simulink model "FourTanks_PID"  (R2023b)
settings: Solver=ode4  StartTime=0.0  StopTime=1600  FixedStep=1/100  MinStep=0.01  RelTol=1e-3  EnableMultiTasking=on
InitFcn:
  | init_fourtanks
model workspace (MAT data in the model file):
  PID_params = [98.4128186329 97.7718380758 37.9597023931 70.0809402327 32.7398112273 96.4014930201]
values from neighbouring files (symbols this model uses):
  A1 = 28    [init_fourtanks.m]
  A2 = 32    [init_fourtanks.m]
  A3 = 28    [init_fourtanks.m]
  A4 = 32    [init_fourtanks.m]
  g = 981    [init_fourtanks.m]
  gamma1 = 0.7    [init_fourtanks.m]
  gamma2 = 0.7    [init_fourtanks.m]
  gamma3 = 1.0    (= 1)    [init_fourtanks.m]
  gamma4 = 1.0    (= 1)    [init_fourtanks.m]
  gammaA = 0.6    [init_fourtanks.m]
  gammaB = 0.6    [init_fourtanks.m]
  k1 = .071    (= 0.071)    [init_fourtanks.m]
  k2 = .057    (= 0.057)    [init_fourtanks.m]
  k3 = .071    (= 0.071)    [init_fourtanks.m]
  k4 = .057    (= 0.057)    [init_fourtanks.m]
  kA = 3.33    [init_fourtanks.m]
  kB = 3.35    [init_fourtanks.m]
undefined symbols (not defined in the file or in its folder): h, sigbuilder_block, u0
libraries: slpidlib x2
settings Model: Creator=Windows  LastModifiedBy=HP
settings SolverCC: AlgebraicLoopSolver=TrustRegion
settings OptimizationCC: DefaultParameterBehavior=Inlined  BufferReuse=off
settings DebuggingCC: UnconnectedInputMsg=warning  UnconnectedOutputMsg=warning  UnconnectedLineMsg=warning  InitInArrayFormatMsg=none  ArithmeticOperatorsInVariantConditions=warning
settings ModelReferenceCC: EnableRefExpFcnMdlSchedulingChecks=on
settings SFSimCC: CustomCodeUndefinedFunction=UseInterfaceOnly
settings RTWCC: DLArmComputeVersion=19.05

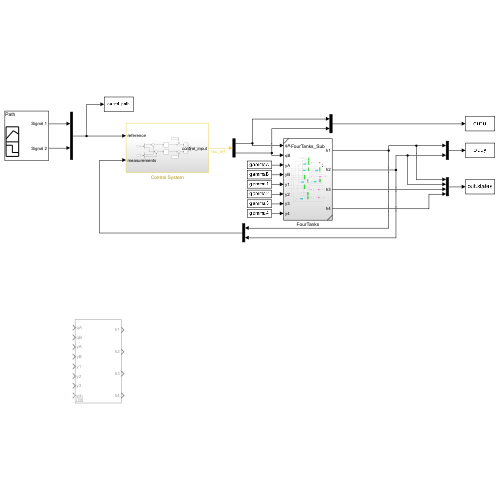
[thumbnail: Simulink's stored preview of the top-level diagram]
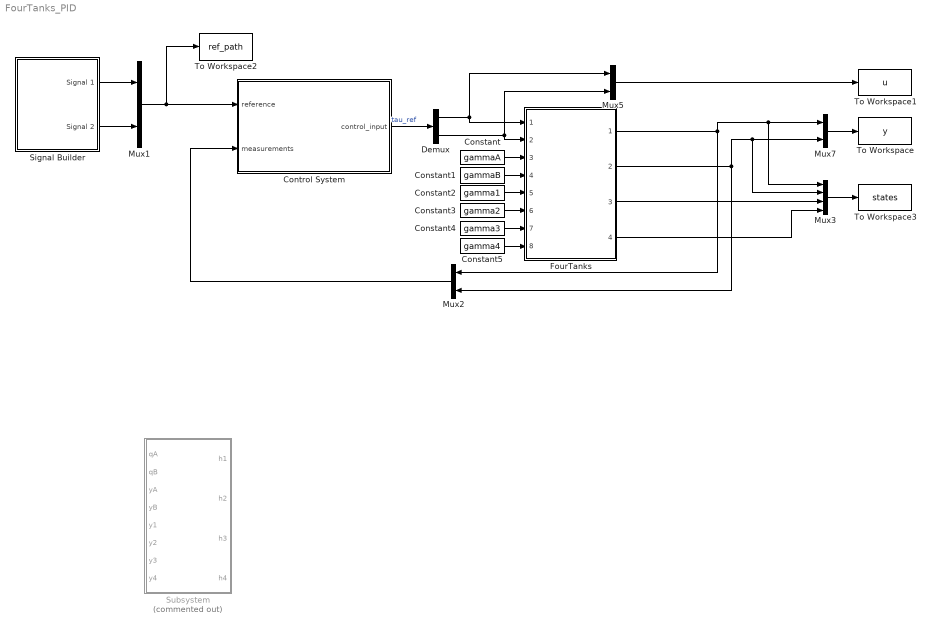
== system FourTanks_PID ==
  Constant : Constant  Value=gammaA
  Constant1 : Constant  Value=gammaB
  Constant2 : Constant  Value=gamma1
  Constant3 : Constant  Value=gamma2
  Constant4 : Constant  Value=gamma3
  Constant5 : Constant  Value=gamma4
  Control System : Subsystem
  Demux : Demux  Outputs=2
  FourTanks : Subsystem  ReferencedSubsystem=FourTanks_Sub
  Mux{1..2,5,7} (4 alike) : Mux  Inputs=2
  Mux3 : Mux
  Signal Builder : Subsystem  Tag=STV Subsys  LoadFcn=sigbuilder_block('load');  StartFcn=sigbuilder_block('start');  StopFcn=sigbuilder_block('stop');  ClipboardFcn=sigbuilder_block('clipboard');  mask(Sigbuilder block){tuvar=[0:10]}
      mask help: Simulink:masks:SigbuilderBlock_MD
      mask init:
      | if ~strcmp(get_param(bdroot(gcbh),'SimulationStatus'),'stopped') tuvar = sigbuilder_block('maskInit'); end
      settings: CopyFcn=sigbuilder_block('copy');  DeleteFcn=sigbuilder_block('delete');  ModelCloseFcn=sigbuilder_block('modelClose');  PreSaveFcn=sigbuilder_block('preSave');  PauseFcn=sigbuilder_block('pause');  ContinueFcn=sigbuilder_block('continue');  NameChangeFcn=sigbuilder_block('namechange');  OpenFcn=sigbuilder_block('open',[5.4 36 1141.2 516.6 ]);  CloseFcn=sigbuilder_block('close');
      mask Display: plot(0, 0, 100, 100,[2, 2, 32, 32, 2], [68, 8, 8, 68, 68],[32, 2], [38, 38], [32, 19, 2],[53, 60, 44], [32, 17, 17, 2],[16, 16, 31, 31]);txt = getActiveGroup(gcbh);text(2, 100, txt,'verticalAlignment', 'top');
  Subsystem : Subsystem  Commented=on
  To Workspace : ToWorkspace  VariableName=y  SaveFormat=Timeseries  SampleTime=-1
      settings: MaxDataPoints=Inf
  To Workspace1 : ToWorkspace  VariableName=u  SaveFormat=Timeseries  SampleTime=-1
      settings: MaxDataPoints=Inf
  To Workspace2 : ToWorkspace  VariableName=ref_path  SaveFormat=Timeseries  SampleTime=-1
      settings: MaxDataPoints=Inf
  To Workspace3 : ToWorkspace  VariableName=states  SaveFormat=Timeseries  SampleTime=-1
      settings: MaxDataPoints=Inf
  wires:
  FourTanks/2 -> Mux2/2, Mux3/2, Mux7/2
  FourTanks/1 -> Mux2/1, Mux3/1, Mux7/1
  Constant1/1 -> FourTanks/4
  Constant2/1 -> FourTanks/5
  Constant3/1 -> FourTanks/6
  Constant4/1 -> FourTanks/7
  Constant5/1 -> FourTanks/8
  Signal Builder/1(Signal 1) -> Mux1/1
  Mux2/1 -> Control System/2(measurements)
  FourTanks/3 -> Mux3/3
  FourTanks/4 -> Mux3/4
  Signal Builder/2(Signal 2) -> Mux1/2
  Mux5/1 -> To Workspace1/1
  Mux7/1 -> To Workspace/1
  Mux3/1 -> To Workspace3/1
  Control System/1(control_input) -> Demux/1  "tau_ref"
  Demux/1 -> FourTanks/1, Mux5/1
  Demux/2 -> FourTanks/2, Mux5/2
  Mux1/1 -> Control System/1(reference), To Workspace2/1
  Constant/1 -> FourTanks/3

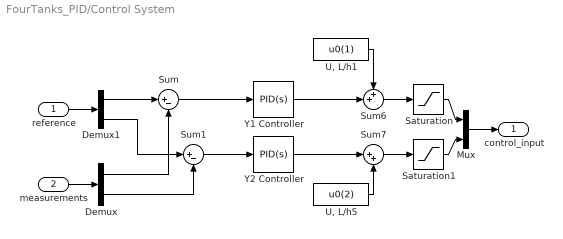
== system FourTanks_PID/Control System ==
  reference : Inport
  measurements : Inport  Port=2
  Demux : Demux  Outputs=2
  Demux1 : Demux  Outputs=2
  Mux : Mux  Inputs=2
  Saturation : Saturate  UpperLimit=3.15  LowerLimit=0
  Saturation1 : Saturate  UpperLimit=3.15  LowerLimit=0
  Sum : Sum  Inputs=|+-
  Sum1 : Sum  Inputs=|+-
  Sum6 : Sum  Inputs=++|
  Sum7 : Sum  Inputs=|++
  "U, L/h1" : Constant  Value=u0(1)
  "U, L/h5" : Constant  Value=u0(2)
  Y1 Controller : slpidlib/PID Controller  Controller=PID  Form=Parallel  TimeDomain=Continuous-time  UseExternalTs=off  SampleTime=-1  IntegratorMethod=Forward Euler  FilterMethod=Forward Euler  ControllerParametersSource=internal  P=PID_params(1)  I=PID_params(2)  UseKiTs=off  D=PID_params(3)  N=100  UseFilter=on  TunerSelectOption=Transfer Function Based (PID Tuner App)  InitialConditionSource=internal  InitialConditionForIntegrator=0  InitialConditionForFilter=0  DifferentiatorICPrevScaledInput=0  ExternalReset=none  TrackingMode=off  Kt=1  LimitOutput=off  SatLimitsSource=internal  UpperSaturationLimit=inf  LowerSaturationLimit=-inf  LinearizeAsGain=on  AntiWindupMode=none  Kb=1  LimitIntegrator=off  UpperIntegratorSaturationLimit=inf  LowerIntegratorSaturationLimit=-inf  POutMin=[]  POutMax=[]  IOutMin=[]  IOutMax=[]  DOutMin=[]  DOutMax=[]  NOutMin=[]  NOutMax=[]  SumOutMin=[]  SumOutMax=[]  SaturationOutMin=[]  SaturationOutMax=[]  PParamMin=[]  PParamMax=[]  IParamMin=[]  IParamMax=[]  DParamMin=[]  DParamMax=[]  NParamMin=[]  NParamMax=[]  KbParamMin=[]  KbParamMax=[]  KtParamMin=[]  KtParamMax=[]  KbOutMin=[]  KbOutMax=[]  KtOutMin=[]  KtOutMax=[]  IntegratorOutMin=[]  IntegratorOutMax=[]  FilterOutMin=[]  FilterOutMax=[]  SumI1OutMin=[]  SumI1OutMax=[]  SumI2OutMin=[]  SumI2OutMax=[]  SumI3OutMin=[]  SumI3OutMax=[]  SumI4OutMin=[]  SumI4OutMax=[]  SumDOutMin=[]  SumDOutMax=[]  DifferentiatorOutMin=[]  DifferentiatorOutMax=[]  FilterDiffOutCoefMin=[]  FilterDiffOutCoefMax=[]  ReciprocalOutMin=[]  ReciprocalOutMax=[]  SumDenOutMin=[]  SumDenOutMax=[]  SumNumOutMin=[]  SumNumOutMax=[]  DivideOutMin=[]  DivideOutMax=[]  UdiffTsProdOutMin=[]  UdiffTsProdOutMax=[]  NTsProdOutMin=[]  NTsProdOutMax=[]  UintegralTsProdOutMin=[]  UintegralTsProdOutMax=[]  UngainTsProdOutMin=[]  UngainTsProdOutMax=[]  ClampingZeroOutDataTypeStr=Inherit: Inherit via back propagation  ClampingZeroOutMin=[]  ClampingZeroOutMax=[]  FilterDenConstantOutDataTypeStr=Inherit: Inherit via back propagation  FilterDenConstantOutMin=[]  FilterDenConstantOutMax=[]  PCopyOutDataTypeStr=Inherit: Inherit via back propagation  PCopyOutMin=[]  PCopyOutMax=[]  NCopyOutDataTypeStr=Inherit: Inherit via back propagation  NCopyOutMin=[]  NCopyOutMax=[]  IntegratorContinuousStateAttributes=''  IntegratorStateMustResolveToSignalObject=off  IntegratorRTWStateStorageClass=Auto  FilterContinuousStateAttributes=''  FilterStateMustResolveToSignalObject=off  FilterRTWStateStorageClass=Auto  ParallelPVariant=InternalParameters  IdealPVariant=Disabled  IVariant=InternalParameters  DVariant=InternalParameters  IntegratorVariant=Continuous  SatVariant=Disabled  AWVariant=Passthrough  PCopyVariant=Disabled  TRVariant=Disabled  FdbkBlocksVariant=Forward  IdealPFdbkVariant=Disabled  SatFdbkVariant=Disabled  DerivativeFilterVariant=ContFilter  NVariant=InternalParameters  NCopyVariant=Disabled  FilterICVariant=InternalICsFilter  IntegratorICVariant=InternalICs  ExternalResetVariant=Disabled  TRSumVariant=Passthrough  SumFdbkVariant=Disabled  SumVariant=Sum_PID  TsampFilterVariant=InternalTs  TsampNgainVariant=Passthrough  TsampIntegralVariant=Disabled_SignalSpec  ExternalSaturationOutDataTypeStr=Inherit: Same as second input
  Y2 Controller : slpidlib/PID Controller  Controller=PID  Form=Parallel  TimeDomain=Continuous-time  UseExternalTs=off  SampleTime=-1  IntegratorMethod=Forward Euler  FilterMethod=Forward Euler  ControllerParametersSource=internal  P=PID_params(4)  I=PID_params(5)  UseKiTs=off  D=PID_params(6)  N=100  UseFilter=on  TunerSelectOption=Transfer Function Based (PID Tuner App)  InitialConditionSource=internal  InitialConditionForIntegrator=0  InitialConditionForFilter=0  DifferentiatorICPrevScaledInput=0  ExternalReset=none  TrackingMode=off  Kt=1  LimitOutput=off  SatLimitsSource=internal  UpperSaturationLimit=inf  LowerSaturationLimit=-inf  LinearizeAsGain=on  AntiWindupMode=none  Kb=1  LimitIntegrator=off  UpperIntegratorSaturationLimit=inf  LowerIntegratorSaturationLimit=-inf  POutMin=[]  POutMax=[]  IOutMin=[]  IOutMax=[]  DOutMin=[]  DOutMax=[]  NOutMin=[]  NOutMax=[]  SumOutMin=[]  SumOutMax=[]  SaturationOutMin=[]  SaturationOutMax=[]  PParamMin=[]  PParamMax=[]  IParamMin=[]  IParamMax=[]  DParamMin=[]  DParamMax=[]  NParamMin=[]  NParamMax=[]  KbParamMin=[]  KbParamMax=[]  KtParamMin=[]  KtParamMax=[]  KbOutMin=[]  KbOutMax=[]  KtOutMin=[]  KtOutMax=[]  IntegratorOutMin=[]  IntegratorOutMax=[]  FilterOutMin=[]  FilterOutMax=[]  SumI1OutMin=[]  SumI1OutMax=[]  SumI2OutMin=[]  SumI2OutMax=[]  SumI3OutMin=[]  SumI3OutMax=[]  SumI4OutMin=[]  SumI4OutMax=[]  SumDOutMin=[]  SumDOutMax=[]  DifferentiatorOutMin=[]  DifferentiatorOutMax=[]  FilterDiffOutCoefMin=[]  FilterDiffOutCoefMax=[]  ReciprocalOutMin=[]  ReciprocalOutMax=[]  SumDenOutMin=[]  SumDenOutMax=[]  SumNumOutMin=[]  SumNumOutMax=[]  DivideOutMin=[]  DivideOutMax=[]  UdiffTsProdOutMin=[]  UdiffTsProdOutMax=[]  NTsProdOutMin=[]  NTsProdOutMax=[]  UintegralTsProdOutMin=[]  UintegralTsProdOutMax=[]  UngainTsProdOutMin=[]  UngainTsProdOutMax=[]  ClampingZeroOutDataTypeStr=Inherit: Inherit via back propagation  ClampingZeroOutMin=[]  ClampingZeroOutMax=[]  FilterDenConstantOutDataTypeStr=Inherit: Inherit via back propagation  FilterDenConstantOutMin=[]  FilterDenConstantOutMax=[]  PCopyOutDataTypeStr=Inherit: Inherit via back propagation  PCopyOutMin=[]  PCopyOutMax=[]  NCopyOutDataTypeStr=Inherit: Inherit via back propagation  NCopyOutMin=[]  NCopyOutMax=[]  IntegratorContinuousStateAttributes=''  IntegratorStateMustResolveToSignalObject=off  IntegratorRTWStateStorageClass=Auto  FilterContinuousStateAttributes=''  FilterStateMustResolveToSignalObject=off  FilterRTWStateStorageClass=Auto  ParallelPVariant=InternalParameters  IdealPVariant=Disabled  IVariant=InternalParameters  DVariant=InternalParameters  IntegratorVariant=Continuous  SatVariant=Disabled  AWVariant=Passthrough  PCopyVariant=Disabled  TRVariant=Disabled  FdbkBlocksVariant=Forward  IdealPFdbkVariant=Disabled  SatFdbkVariant=Disabled  DerivativeFilterVariant=ContFilter  NVariant=InternalParameters  NCopyVariant=Disabled  FilterICVariant=InternalICsFilter  IntegratorICVariant=InternalICs  ExternalResetVariant=Disabled  TRSumVariant=Passthrough  SumFdbkVariant=Disabled  SumVariant=Sum_PID  TsampFilterVariant=InternalTs  TsampNgainVariant=Passthrough  TsampIntegralVariant=Disabled_SignalSpec  ExternalSaturationOutDataTypeStr=Inherit: Same as second input
  control_input : Outport  VectorParamsAs1DForOutWhenUnconnected=off
  wires:
  Sum/1 -> Y1 Controller/1
  Sum1/1 -> Y2 Controller/1
  measurements/1 -> Demux/1
  Demux/1 -> Sum/2
  Demux/2 -> Sum1/2
  reference/1 -> Demux1/1
  Demux1/1 -> Sum/1
  Demux1/2 -> Sum1/1
  Y1 Controller/1 -> Sum6/2
  Sum7/1 -> Saturation1/1
  "U, L/h1"/1 -> Sum6/1
  Sum6/1 -> Saturation/1
  "U, L/h5"/1 -> Sum7/2
  Y2 Controller/1 -> Sum7/1
  Saturation/1 -> Mux/1
  Saturation1/1 -> Mux/2
  Mux/1 -> control_input/1

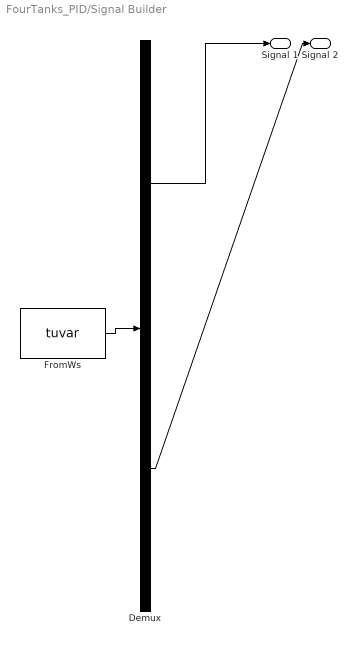
== system FourTanks_PID/Signal Builder ==
  Demux : Demux  Tag=STV Demux  Outputs=2
      settings: DisplayOption=none
  FromWs : FromWorkspace  Tag=STV FromWs  VariableName=tuvar
      SigBuilderData=|
      | common.afterFinalStr = 'Extrapolate'
      | common.sampleTime = 0
      | dataSet(1).timeRange = [0 1600]
      | dataSet(1).name = 'Path'
      | dataSet(2).timeRange = [0 1600]
      | dataSet(2).name = 'Step1'
      | dataSet(3).timeRange = [0 1600]
      | dataSet(3).name = 'Step2'
      | sbobj.Groups(1).Name = 'Path'
      | sbobj.Groups(1).Signals(1).Name = 'Signal 1'
      | sbobj.Groups(1).Signals(1).XData = [0 700 700 1200 1200 1600]
      | sbobj.Groups(1).Signals(1).YData = [12.75 12.75 11.5 11.5 11 11]
      | sbobj.Groups(1).Signals(2).Name = 'Signal 2'
      | sbobj.Groups(1).Signals(2).XData = [0 400 400 1200 1200 1600]
      | sbobj.Groups(1).Signals(2).YData = [12.8 12.8 11.5 11.5 12 12]
      | sbobj.Groups(1).TimeRange = [0 1600]
      | sbobj.Groups(2).Name = 'Step1'
      | sbobj.Groups(2).Signals(1).Name = 'Signal 1'
      | sbobj.Groups(2).Signals(1).XData = [0 200 200 1200 1600]
      | sbobj.Groups(2).Signals(1).YData = [12.75 12.75 11.5 11.5 11.5]
      | sbobj.Groups(2).Signals(2).Name = 'Signal 2'
      | sbobj.Groups(2).Signals(2).XData = [0 400 1200 1600]
      | sbobj.Groups(2).Signals(2).YData = [12.8 12.8 12.8 12.8]
      | sbobj.Groups(2).TimeRange = [0 1600]
      | sbobj.Groups(3).Name = 'Step2'
      | sbobj.Groups(3).Signals(1).Name = 'Signal 1'
      | sbobj.Groups(3).Signals(1).XData = [0 200 1200 1600]
      | sbobj.Groups(3).Signals(1).YData = [12.75 12.75 12.75 12.75]
      | sbobj.Groups(3).Signals(2).Name = 'Signal 2'
      | sbobj.Groups(3).Signals(2).XData = [0 200 200 1600]
      | sbobj.Groups(3).Signals(2).YData = [12.8 12.8 11.5 11.5]
      | sbobj.Groups(3).TimeRange = [0 1600]
  Signal 1 : Outport  Tag=STV Outport  VectorParamsAs1DForOutWhenUnconnected=off
  Signal 2 : Outport  Tag=STV Outport  Port=2  VectorParamsAs1DForOutWhenUnconnected=off
  wires:
  Demux/1 -> Signal 1/1
  FromWs/1 -> Demux/1
  Demux/2 -> Signal 2/1

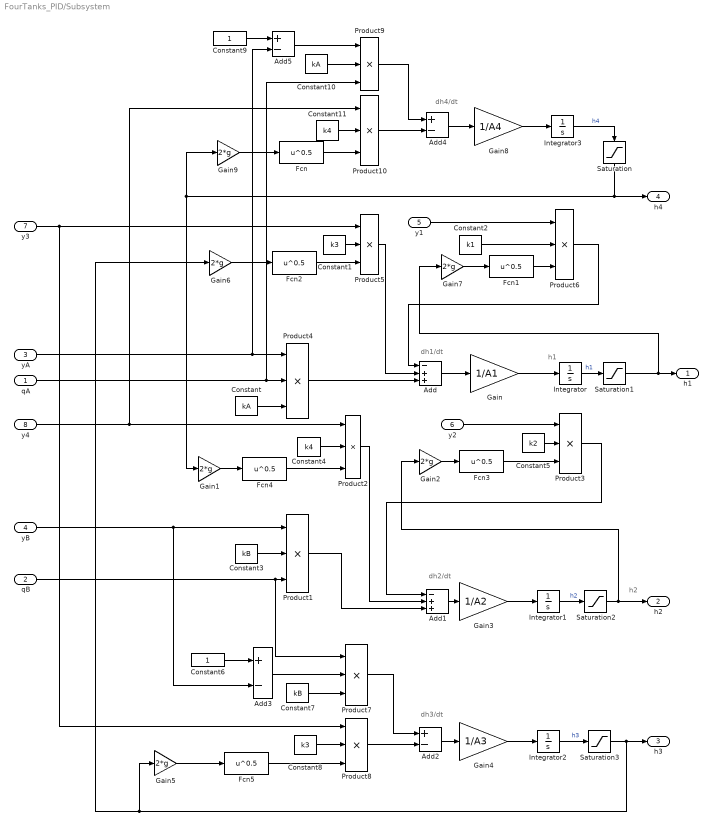
== system FourTanks_PID/Subsystem ==
  note: h2
  note: dh2/dt
  note: dh1/dt
  note: h1
  note: dh3/dt
  note: dh4/dt
  qA : Inport
  qB : Inport  Port=2
  yA : Inport  Port=3
  yB : Inport  Port=4
  y1 : Inport  Port=5
  y2 : Inport  Port=6
  y3 : Inport  Port=7
  y4 : Inport  Port=8
  Add : Sum  Inputs=-++
  Add1 : Sum  Inputs=-++
  Add{2..5} (4 alike) : Sum  Inputs=+-
  Constant : Constant  Value=kA
  Constant1 : Constant  Value=k3
  Constant10 : Constant  Value=kA
  Constant11 : Constant  Value=k4
  Constant2 : Constant  Value=k1
  Constant3 : Constant  Value=kB
  Constant4 : Constant  Value=k4
  Constant5 : Constant  Value=k2
  Constant6 : Constant
  Constant7 : Constant  Value=kB
  Constant8 : Constant  Value=k3
  Constant9 : Constant
  Fcn{,1..5} (6 alike) : Fcn  Expr=u^0.5
  Gain : Gain  Gain=1/A1
  Gain{1..2,5..7,9} (6 alike) : Gain  Gain=2*g
  Gain3 : Gain  Gain=1/A2
  Gain4 : Gain  Gain=1/A3
  Gain8 : Gain  Gain=1/A4
  Integrator : Integrator  InitialCondition=h(1)
  Integrator1 : Integrator  InitialCondition=h(2)
  Integrator2 : Integrator  InitialCondition=h(3)
  Integrator3 : Integrator  InitialCondition=h(4)
  Product{1..10} (10 alike) : Product  Inputs=3  RndMeth=Zero
  Saturation{,1..3} (4 alike) : Saturate  UpperLimit=inf  LowerLimit=0
  h1 : Outport
  h2 : Outport  Port=2
  h3 : Outport  Port=3
  h4 : Outport  Port=4
  wires:
  Constant3/1 -> Product1/2
  Integrator/1 -> Saturation1/1  "h1"
  Integrator2/1 -> Saturation3/1  "h3"
  y3/1 -> Product8/1, Product5/1
  Constant10/1 -> Product9/2
  Constant8/1 -> Product8/2
  Integrator1/1 -> Saturation2/1  "h2"
  Gain8/1 -> Integrator3/1
  Integrator3/1 -> Saturation/1  "h4"
  y4/1 -> Product10/1, Product2/1
  qA/1 -> Product9/3, Product4/2
  Product9/1 -> Add4/1
  Fcn1/1 -> Product6/3
  Constant11/1 -> Product10/2
  Add3/1 -> Product7/2
  Gain2/1 -> Fcn3/1
  Fcn4/1 -> Product2/3
  Constant6/1 -> Add3/1
  Constant5/1 -> Product3/2
  Gain3/1 -> Integrator1/1
  Product10/1 -> Add4/2
  Constant7/1 -> Product7/3
  Gain6/1 -> Fcn2/1
  Constant9/1 -> Add5/1
  Add5/1 -> Product9/1
  yA/1 -> Add5/2, Product4/1
  Gain5/1 -> Fcn5/1
  qB/1 -> Product7/1, Product1/3
  Fcn2/1 -> Product5/3
  Add4/1 -> Gain8/1
  Fcn5/1 -> Product8/3
  Product7/1 -> Add2/1
  Gain/1 -> Integrator/1
  Gain4/1 -> Integrator2/1
  Product3/1 -> Add1/1
  Constant2/1 -> Product6/2
  Product2/1 -> Add1/2
  Product1/1 -> Add1/3
  Gain1/1 -> Fcn4/1
  Add2/1 -> Gain4/1
  y2/1 -> Product3/1
  Product8/1 -> Add2/2
  Gain9/1 -> Fcn/1
  Constant/1 -> Product4/3
  y1/1 -> Product6/1
  Constant1/1 -> Product5/2
  Product5/1 -> Add/2
  Constant4/1 -> Product2/2
  Add/1 -> Gain/1
  yB/1 -> Add3/2, Product1/1
  Fcn/1 -> Product10/3
  Add1/1 -> Gain3/1
  Product4/1 -> Add/3
  Gain7/1 -> Fcn1/1
  Fcn3/1 -> Product3/3
  Product6/1 -> Add/1
  Saturation/1 -> Gain1/1, Gain9/1, h4/1
  Saturation1/1 -> h1/1, Gain7/1
  Saturation2/1 -> Gain2/1, h2/1
  Saturation3/1 -> h3/1, Gain5/1, Gain6/1
